simulink model "Model"  (R2020b)
settings: Solver=VariableStepAuto  StartTime=0.0  StopTime=20  MaxStep=0.1  RelTol=1e-1
values from neighbouring files (symbols this model uses):
  D = [0 ... (first row only)    [Data_clean.m]
  g = 9.81    [Data_clean.m]
  k_cart = 0.0113    [Data_clean.m]
  L = 5    [Data_clean.m]
  m = 12000    [Data_clean.m]
  M = 1000    [Data_clean.m]
  Ts = 0.1    [Data_clean.m]
undefined symbols (not defined in the file or in its folder): blk, Discrete, iA, isLTV, lastPcov, lastu, lastx, MDscale, mpc1_plant, MVscale, nCC, nu, nud, nv, nxp, ny, nym, p, RMVscale, Time, ts, uoff, X, xoff, Y, Yscale, Z
libraries: sm_lib x76, mpcsigdimcheck_private x76, nesl_utility x12, ctrlSharedLib x8, simulink_extras x5, mpclib x1
(part 6 of 8)

== system Model/Adaptive MPC Controller2/MPC/MPC Matrix Signal Check U ==
  Input : Inport
  Matrix Dimension Check : S-Function  FunctionName=mpcMatrixSignalCheck  Parameters=blockname, signalname, nrow, ncol, nsteps, isltv  SFunctionDeploymentMode=off  EnableBusSupport=off
  Signal Specification : SignalSpecification  Dimensions=[1 1]
  Output : Outport  VectorParamsAs1DForOutWhenUnconnected=off
  wires:
  Input/1 -> Output/1, Signal Specification/1
  Signal Specification/1 -> Matrix Dimension Check/1

== system Model/Adaptive MPC Controller2/MPC/MPC Matrix Signal Check X ==
  Input : Inport
  Matrix Dimension Check : S-Function  FunctionName=mpcMatrixSignalCheck  Parameters=blockname, signalname, nrow, ncol, nsteps, isltv  SFunctionDeploymentMode=off  EnableBusSupport=off
  Signal Specification : SignalSpecification  Dimensions=[4 1]
  Output : Outport  VectorParamsAs1DForOutWhenUnconnected=off
  wires:
  Input/1 -> Output/1, Signal Specification/1
  Signal Specification/1 -> Matrix Dimension Check/1

== system Model/Adaptive MPC Controller2/MPC/MPC Matrix Signal Check Y ==
  Input : Inport
  Matrix Dimension Check : S-Function  FunctionName=mpcMatrixSignalCheck  Parameters=blockname, signalname, nrow, ncol, nsteps, isltv  SFunctionDeploymentMode=off  EnableBusSupport=off
  Signal Specification : SignalSpecification  Dimensions=[4 1]
  Output : Outport  VectorParamsAs1DForOutWhenUnconnected=off
  wires:
  Input/1 -> Output/1, Signal Specification/1
  Signal Specification/1 -> Matrix Dimension Check/1

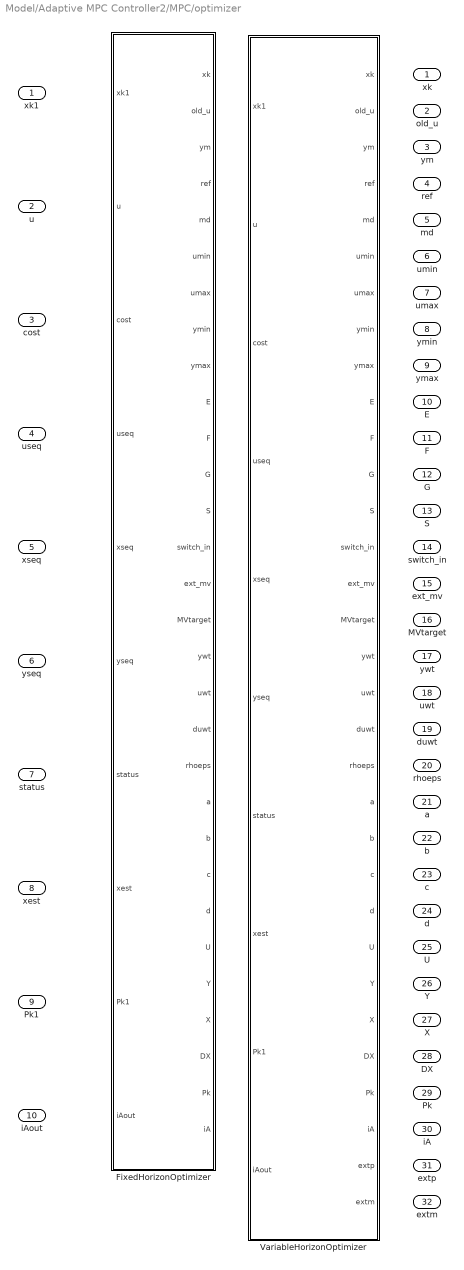
== system Model/Adaptive MPC Controller2/MPC/optimizer ==
  "xk " : Inport
  "old_u " : Inport  Port=2
  "ym " : Inport  Port=3
  "ref " : Inport  Port=4
  "md " : Inport  Port=5
  "umin " : Inport  Port=6
  "umax " : Inport  Port=7
  "ymin " : Inport  Port=8
  "ymax " : Inport  Port=9
  "E " : Inport  Port=10
  "F " : Inport  Port=11
  "G " : Inport  Port=12
  "S " : Inport  Port=13
  "switch_in " : Inport  Port=14
  "ext_mv " : Inport  Port=15
  "MVtarget " : Inport  Port=16
  "ywt " : Inport  Port=17
  "uwt " : Inport  Port=18
  "duwt " : Inport  Port=19
  "rhoeps " : Inport  Port=20
  "a " : Inport  Port=21
  "b " : Inport  Port=22
  "c " : Inport  Port=23
  "d " : Inport  Port=24
  "U " : Inport  Port=25
  "Y " : Inport  Port=26
  "X " : Inport  Port=27
  "DX " : Inport  Port=28
  "Pk " : Inport  Port=29
  "iA " : Inport  Port=30
  extp : Inport  Port=31
  extm : Inport  Port=32
  FixedHorizonOptimizer : MATLAB Function  VariantControl=FixedHorizon
  VariableHorizonOptimizer : MATLAB Function  VariantControl=VariableHorizon
  " xk1" : Outport  VectorParamsAs1DForOutWhenUnconnected=off
  " u" : Outport  Port=2  VectorParamsAs1DForOutWhenUnconnected=off
  " cost" : Outport  Port=3  VectorParamsAs1DForOutWhenUnconnected=off
  " useq" : Outport  Port=4  VectorParamsAs1DForOutWhenUnconnected=off
  " xseq" : Outport  Port=5  VectorParamsAs1DForOutWhenUnconnected=off
  " yseq" : Outport  Port=6  VectorParamsAs1DForOutWhenUnconnected=off
  " status" : Outport  Port=7  VectorParamsAs1DForOutWhenUnconnected=off
  " xest" : Outport  Port=8  VectorParamsAs1DForOutWhenUnconnected=off
  " Pk1" : Outport  Port=9  VectorParamsAs1DForOutWhenUnconnected=off
  " iAout" : Outport  Port=10  VectorParamsAs1DForOutWhenUnconnected=off

== system Model/Adaptive MPC Controller3/MPC/MPC Matrix Signal Check A ==
  Input : Inport
  Matrix Dimension Check : S-Function  FunctionName=mpcMatrixSignalCheck  Parameters=blockname, signalname, nrow, ncol, nsteps, isltv  SFunctionDeploymentMode=off  EnableBusSupport=off
  Signal Specification : SignalSpecification  Dimensions=[4 4]
  Output : Outport  VectorParamsAs1DForOutWhenUnconnected=off
  wires:
  Input/1 -> Output/1, Signal Specification/1
  Signal Specification/1 -> Matrix Dimension Check/1

== system Model/Adaptive MPC Controller3/MPC/MPC Matrix Signal Check B ==
  Input : Inport
  Matrix Dimension Check : S-Function  FunctionName=mpcMatrixSignalCheck  Parameters=blockname, signalname, nrow, ncol, nsteps, isltv  SFunctionDeploymentMode=off  EnableBusSupport=off
  Signal Specification : SignalSpecification  Dimensions=[4 1]
  Output : Outport  VectorParamsAs1DForOutWhenUnconnected=off
  wires:
  Input/1 -> Output/1, Signal Specification/1
  Signal Specification/1 -> Matrix Dimension Check/1

== system Model/Adaptive MPC Controller3/MPC/MPC Matrix Signal Check C ==
  Input : Inport
  Matrix Dimension Check : S-Function  FunctionName=mpcMatrixSignalCheck  Parameters=blockname, signalname, nrow, ncol, nsteps, isltv  SFunctionDeploymentMode=off  EnableBusSupport=off
  Signal Specification : SignalSpecification  Dimensions=[4 4]
  Output : Outport  VectorParamsAs1DForOutWhenUnconnected=off
  wires:
  Input/1 -> Output/1, Signal Specification/1
  Signal Specification/1 -> Matrix Dimension Check/1

== system Model/Adaptive MPC Controller3/MPC/MPC Matrix Signal Check D ==
  Input : Inport
  Matrix Dimension Check : S-Function  FunctionName=mpcMatrixSignalCheck  Parameters=blockname, signalname, nrow, ncol, nsteps, isltv  SFunctionDeploymentMode=off  EnableBusSupport=off
  Signal Specification : SignalSpecification  Dimensions=[4 1]
  Output : Outport  VectorParamsAs1DForOutWhenUnconnected=off
  wires:
  Input/1 -> Output/1, Signal Specification/1
  Signal Specification/1 -> Matrix Dimension Check/1

== system Model/Adaptive MPC Controller3/MPC/MPC Matrix Signal Check DX ==
  Input : Inport
  Matrix Dimension Check : S-Function  FunctionName=mpcMatrixSignalCheck  Parameters=blockname, signalname, nrow, ncol, nsteps, isltv  SFunctionDeploymentMode=off  EnableBusSupport=off
  Signal Specification : SignalSpecification  Dimensions=[4 1]
  Output : Outport  VectorParamsAs1DForOutWhenUnconnected=off
  wires:
  Input/1 -> Output/1, Signal Specification/1
  Signal Specification/1 -> Matrix Dimension Check/1

== system Model/Adaptive MPC Controller3/MPC/MPC Matrix Signal Check U ==
  Input : Inport
  Matrix Dimension Check : S-Function  FunctionName=mpcMatrixSignalCheck  Parameters=blockname, signalname, nrow, ncol, nsteps, isltv  SFunctionDeploymentMode=off  EnableBusSupport=off
  Signal Specification : SignalSpecification  Dimensions=[1 1]
  Output : Outport  VectorParamsAs1DForOutWhenUnconnected=off
  wires:
  Input/1 -> Output/1, Signal Specification/1
  Signal Specification/1 -> Matrix Dimension Check/1

== system Model/Adaptive MPC Controller3/MPC/MPC Matrix Signal Check X ==
  Input : Inport
  Matrix Dimension Check : S-Function  FunctionName=mpcMatrixSignalCheck  Parameters=blockname, signalname, nrow, ncol, nsteps, isltv  SFunctionDeploymentMode=off  EnableBusSupport=off
  Signal Specification : SignalSpecification  Dimensions=[4 1]
  Output : Outport  VectorParamsAs1DForOutWhenUnconnected=off
  wires:
  Input/1 -> Output/1, Signal Specification/1
  Signal Specification/1 -> Matrix Dimension Check/1

== system Model/Adaptive MPC Controller3/MPC/MPC Matrix Signal Check Y ==
  Input : Inport
  Matrix Dimension Check : S-Function  FunctionName=mpcMatrixSignalCheck  Parameters=blockname, signalname, nrow, ncol, nsteps, isltv  SFunctionDeploymentMode=off  EnableBusSupport=off
  Signal Specification : SignalSpecification  Dimensions=[4 1]
  Output : Outport  VectorParamsAs1DForOutWhenUnconnected=off
  wires:
  Input/1 -> Output/1, Signal Specification/1
  Signal Specification/1 -> Matrix Dimension Check/1

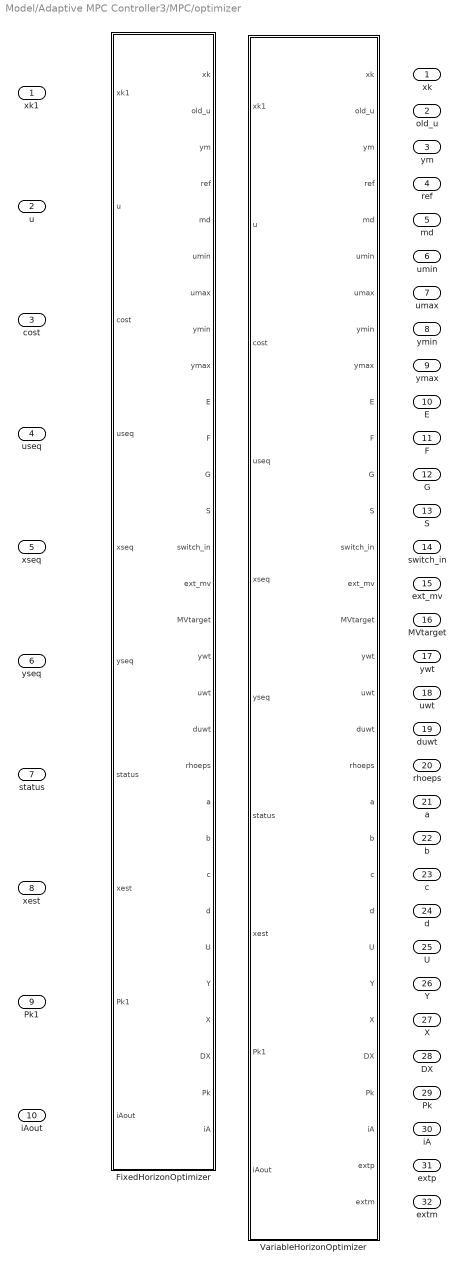
== system Model/Adaptive MPC Controller3/MPC/optimizer ==
  "xk " : Inport
  "old_u " : Inport  Port=2
  "ym " : Inport  Port=3
  "ref " : Inport  Port=4
  "md " : Inport  Port=5
  "umin " : Inport  Port=6
  "umax " : Inport  Port=7
  "ymin " : Inport  Port=8
  "ymax " : Inport  Port=9
  "E " : Inport  Port=10
  "F " : Inport  Port=11
  "G " : Inport  Port=12
  "S " : Inport  Port=13
  "switch_in " : Inport  Port=14
  "ext_mv " : Inport  Port=15
  "MVtarget " : Inport  Port=16
  "ywt " : Inport  Port=17
  "uwt " : Inport  Port=18
  "duwt " : Inport  Port=19
  "rhoeps " : Inport  Port=20
  "a " : Inport  Port=21
  "b " : Inport  Port=22
  "c " : Inport  Port=23
  "d " : Inport  Port=24
  "U " : Inport  Port=25
  "Y " : Inport  Port=26
  "X " : Inport  Port=27
  "DX " : Inport  Port=28
  "Pk " : Inport  Port=29
  "iA " : Inport  Port=30
  extp : Inport  Port=31
  extm : Inport  Port=32
  FixedHorizonOptimizer : MATLAB Function  VariantControl=FixedHorizon
  VariableHorizonOptimizer : MATLAB Function  VariantControl=VariableHorizon
  " xk1" : Outport  VectorParamsAs1DForOutWhenUnconnected=off
  " u" : Outport  Port=2  VectorParamsAs1DForOutWhenUnconnected=off
  " cost" : Outport  Port=3  VectorParamsAs1DForOutWhenUnconnected=off
  " useq" : Outport  Port=4  VectorParamsAs1DForOutWhenUnconnected=off
  " xseq" : Outport  Port=5  VectorParamsAs1DForOutWhenUnconnected=off
  " yseq" : Outport  Port=6  VectorParamsAs1DForOutWhenUnconnected=off
  " status" : Outport  Port=7  VectorParamsAs1DForOutWhenUnconnected=off
  " xest" : Outport  Port=8  VectorParamsAs1DForOutWhenUnconnected=off
  " Pk1" : Outport  Port=9  VectorParamsAs1DForOutWhenUnconnected=off
  " iAout" : Outport  Port=10  VectorParamsAs1DForOutWhenUnconnected=off

== matlab function Model/Plant Model3 ==
  data: u input; A output; x input; B output; C output; D output; U output; Y output; X output; DX output; m input; L input
function [A,B,C,D,U,Y,X,DX] = fcn(u,x,m,L)
% Sample time
Ts = 0.1;

% Model parameters
M = 1000;               % Cart mass, kg
g = 9.81;               % Gravity constant, m/s^2 
k_cart = 0.0113;        % Rolling resistance coefficient   

% Continuos-time model
% Calculated constants
c1 = 1 - m/(m + M);
c2 = -1/(L*(m + M));

A = [-k_cart*(m + M)*g/M    0     0    m*g/M
              1             0     0      0
       k_cart*g/(L*c1)      0     0  -g/(L*c1) 
              0             0     1      0];
 
B = [1/M
      0
    c2/c1
      0];

C = [0 1 0 0
     1 0 0 0
     0 0 0 1
     0 0 1 0];
     
D = [0
     0
     0
     0];
  
% Generate discrete-time model
nx = size(A,1);
nu = size(B,2);
Mr = expm([[A B]*Ts; zeros(nu,nx+nu)]);
A = Mr(1:nx,1:nx);
B = Mr(1:nx,nx+1:nx+nu);

% Nominal conditions for discrete-time plant
X = x;
U = u;
Y = C*x + D*u;
DX = A*x+B*u-x;

== matlab function Model/no_expm1 ==
  data: u input; A output; x input; B output; C output; D output; U output; Y output; X output; DX output; m input; L input
function [A,B,C,D,U,Y,X,DX] = fcn(u,x,m,L)
% Sample time
Ts = 0.1;

% Model parameters
M = 1000;               % Cart mass, kg
g = 9.81;               % Gravity constant, m/s^2 
k_cart = 0.0113;        % Rolling resistance coefficient   

% Continuos-time model
% Calculated constants
c1 = 1 - m/(m + M);
c2 = -1/(L*(m + M));

Ac = [-k_cart*(m + M)*g/M    0     0    m*g/M
              1              0     0      0
       k_cart*g/(L*c1)       0     0  -g/(L*c1) 
              0              0     1      0];
 
Bc = [1/M
       0
     c2/c1
       0];

Cc = [0 1 0 0
      1 0 0 0
      0 0 0 1
      0 0 1 0];
     
Dc = [0
      0
      0
      0];
  
% Generate discrete-time model
nx = size(Ac,1);
nu = size(Bc,2);

% Expm function
X_exp = [[Ac Bc]*Ts; zeros(nu,nx+nu)];
[V_exp,D_exp] = eig(X_exp);
Mr = real(V_exp*diag(exp(diag(D_exp)))/V_exp);
Mr(2,5) = 0;

A = Mr(1:nx,1:nx);
B = Mr(1:nx,nx+1:nx+nu);

% Nominal conditions for discrete-time plant
C = Cc;
D = Dc;

X = x;
U = u;
Y = C*x + D*u;
DX = A*x+B*u-x;

== matlab function Model/Adaptive MPC Controller3/MPC/optimizer/FixedHorizonOptimizer ==
  settings: updateMethod=DISCRETE  sampleTime=ts
  data: xk1 output BlockDataType; xk input BlockDataType; old_u input BlockDataType; ym input BlockDataType; ref input BlockDataType; md input BlockDataType; umin input BlockDataType; umax input BlockDataType; ymin input BlockDataType; ymax input BlockDataType; E input BlockDataType; F input BlockDataType; G input BlockDataType; S input BlockDataType; switch_in input BlockDataType; ext_mv input BlockDataType; MVtarget input BlockDataType; isQP parameter boolean; nx parameter BlockDataType; nxp parameter BlockDataType; nup parameter BlockDataType; nu parameter BlockDataType; ny parameter BlockDataType; degrees parameter BlockDataType; Hinv parameter BlockDataType; Kx parameter BlockDataType; Ku1 parameter BlockDataType; Kut parameter BlockDataType; Kr parameter BlockDataType; Kv parameter BlockDataType; Mlim parameter BlockDataType; Mx parameter BlockDataType; Mu1 parameter BlockDataType; Mv parameter BlockDataType; z_degrees parameter BlockDataType; utarget parameter BlockDataType; p parameter BlockDataType; CustomSolver parameter boolean; CustomSolverCodeGen parameter boolean; UseSuboptimalSolution parameter boolean; UseActiveSetSolver parameter boolean; ASOptions parameter; nxQP parameter BlockDataType; openloopflag parameter boolean; no_umin parameter BlockDataType; no_umax parameter BlockDataType; no_ymin parameter BlockDataType; no_ymax parameter BlockDataType; switch_inport parameter BlockDataType; no_switch parameter BlockDataType; enable_value parameter BlockDataType; return_cost parameter BlockDataType; H parameter BlockDataType; return_mvseq parameter BlockDataType; return_xseq parameter BlockDataType; return_ovseq parameter BlockDataType; Linv parameter BlockDataType; Ac parameter BlockDataType; ywt input BlockDataType; uwt input BlockDataType; duwt input BlockDataType; rhoeps input BlockDataType; isLTV parameter boolean; a input BlockDataType; b input BlockDataType; c input BlockDataType; d input BlockDataType; U input BlockDataType; Y input BlockDataType; X input BlockDataType; DX input BlockDataType; Pk input BlockDataType; iA input boolean; u output BlockDataType; cost output BlockDataType; useq output BlockDataType; xseq output BlockDataType; yseq output BlockDataType; status output BlockDataType; xest output BlockDataType; Pk1 output BlockDataType; no_ywt parameter BlockDataType; no_uwt parameter BlockDataType; no_duwt parameter BlockDataType; no_rhoeps parameter BlockDataType; Wy parameter BlockDataType; Wdu parameter BlockDataType; Jm parameter BlockDataType; SuJm parameter BlockDataType; Su1 parameter BlockDataType; Sx parameter BlockDataType; Hv parameter BlockDataType; Wu parameter BlockDataType; I1 parameter BlockDataType; iAout output boolean; A parameter BlockDataType; C parameter BlockDataType; B parameter BlockDataType; D parameter BlockDataType; Cid parameter BlockDataType; Did parameter BlockDataType; Mrows parameter BlockDataType; nCC parameter BlockDataType; Ecc parameter BlockDataType; Fcc parameter BlockDataType; Scc parameter BlockDataType; Gcc parameter BlockDataType; nv parameter BlockDataType; no_md parameter BlockDataType; no_ref parameter BlockDataType; no_uref parameter BlockDataType; no_mv parameter BlockDataType; RYscale parameter BlockDataType; RMDscale parameter BlockDataType; myindex parameter BlockDataType; xoff parameter BlockDataType; CustomEstimation parameter boolean; mvindex parameter BlockDataType; mdindex parameter BlockDataType; unindex parameter BlockDataType; nxid parameter BlockDataType; Uscale parameter BlockDataType; Yscale parameter BlockDataType; uoff parameter BlockDataType; voff parameter BlockDataType; yoff parameter BlockDataType; myoff parameter BlockDataType; no_cc parameter BlockDataType; IPOptions parameter; RMVscale parameter; m parameter
function [xk1, u, cost, useq, xseq, yseq, status, xest, Pk1, iAout] = fcn(...
            xk, old_u, ym, ref, md, umin, umax, ymin, ymax, E, F, G, S,...
            switch_in, ext_mv, MVtarget, isQP, nx, nxp, nup, ...
            nu, ny, degrees, Hinv, Kx, Ku1, Kut, Kr, Kv, Mlim, ...
            Mx, Mu1, Mv, z_degrees, utarget, p, ...
            CustomSolver, CustomSolverCodeGen, UseSuboptimalSolution, ...
            UseActiveSetSolver, ASOptions, nxQP, openloopflag, ...
            no_umin, no_umax, no_ymin, no_ymax, switch_inport, no_switch, enable_value, ...
            return_cost, H, return_mvseq, return_xseq, return_ovseq, Linv, Ac, ...
            ywt, uwt, duwt, rhoeps, isLTV, a, b, c, d, U, Y, X, DX, Pk, iA, ...
            no_ywt, no_uwt, no_duwt, no_rhoeps,...
            Wy, Wdu, Jm, SuJm, Su1, Sx, Hv, Wu, I1, ...
            A, C, B, D, Cid, Did, Mrows, nCC, Ecc, Fcc, Scc, Gcc, ...
            nv, no_md, no_ref, no_uref, no_mv, RYscale, RMDscale, myindex, ...
            xoff, CustomEstimation, mvindex, mdindex, unindex, nxid, Uscale, Yscale, uoff, voff, yoff, myoff, no_cc, IPOptions, RMVscale, m)
%#codegen
coder.extrinsic('mpcblock_optimizer_double_mex');
coder.extrinsic('mpcblock_optimizer_single_mex');
coder.extrinsic('mpcblock_refmd_double_mex');
coder.extrinsic('mpcblock_refmd_single_mex');

% Constants
isSimulation = coder.target('Sfun') && ~coder.target('RtwForRapid') && ~coder.target('RtwForSim');
isAdaptive = ~isLTV; % isLTV=true forces isAdaptive=false
isDouble = isa(ref,'double');
if isDouble
    DataType = 'double';
else
    DataType = 'single';
end
ZERO = zeros('like',ref);
ONE = ones('like',ref);
hasMD = nv>1;

% Pre-allocate all the MEX block outputs for the simulation mode
%#ok<*NASGU>
if isSimulation
    rseq = zeros(p*ny,1,'like',ref); %#ok<*NASGU>
    vseq = zeros((p+1)*nv,1,'like',ref);
    v = zeros(nv,1,'like',ref);
    xk1 = zeros(nx,1,'like',ref);
    u = zeros(nu,1,'like',ref);
    cost = ZERO;
    useq = zeros(p+1,nu,'like',ref); %#ok<*PREALL>
    status = ONE;
    xest = zeros(nx,1,'like',ref);
    iAout = iA;
end

% Model update
nym = length(myindex);
ai=zeros(nxp,nxp,'like',ref);
bi=zeros(nxp,nup,'like',ref);
ci=zeros(ny,nxp,'like',ref);
di=zeros(ny,nup,'like',ref);

ai(:,:)=a(:,:,1);
bi(:,:)=b(:,:,1);
ci(:,:)=c(:,:,1);
di(:,:)=d(:,:,1);

% Allocate matrices. Must allocate 3D matrix also in Adaptive case,
% otherwise EML code does not compile.
Bu=zeros(nx,nu,p+1,'like',ref);
Bv=zeros(nx,nv,p+1,'like',ref);
Dv=zeros(ny,nv,p+1,'like',ref);
Dvm=zeros(nym,nv,p+1,'like',ref);
Cm=zeros(nym,nx,p+1,'like',ref);
if ~isLTV
    % Adaptive
    [A(:,:,1),C(:,:,1),Bu(:,:,1),Bv(:,:,1),Cm(:,:,1),Dv(:,:,1),Dvm(:,:,1),Qk,Rk,Nk] = mpc_plantupdate(...
        ai,bi,ci,di,A(:,:,1),B(:,:,1),C(:,:,1),D(:,:,1),mvindex,mdindex,unindex,nxp,nup,ny,nv,nxid, ...
        myindex,Uscale,Yscale,Cid,Did);
else
    % Retrieve LTV model
    for i=1:p+1
        ai(1:nxp,1:nxp)=a(:,:,i);
        bi(1:nxp,1:nup)=b(:,:,i);
        ci(1:ny,1:nxp)=c(:,:,i);
        di(1:ny,1:nup)=d(:,:,i);
        [A(:,:,i),C(:,:,i),Bu(:,:,i),Bv(:,:,i),Cm(:,:,i),Dv(:,:,i),Dvm(:,:,i),Qk,Rk,Nk] =...
            mpc_plantupdate(ai,bi,ci,di,A(:,:,i),B(:,:,i),C(:,:,i),D(:,:,i),mvindex,mdindex,unindex,nxp,nup,ny,nv,nxid, ...
            myindex,Uscale,Yscale,Cid,Did);
    end
end

% Offset update together with Mlim, utarget, Bv and Dv values
[Mlim, utarget, uoff, voff, yoff, myoff, xoff, Bv, Dv] = ...
    mpc_updateFromNominal(isAdaptive,isQP,p,Mlim,Mrows,...
       U,Uscale,uoff,mvindex,voff,mdindex,utarget,nu,nv-1,...
       Y,Yscale,yoff,myoff,myindex,ny,...
       X,xoff,nxp,DX,A,Bu,Bv,C,Dv,nCC);

% Remove last u offset
old_u = old_u - uoff;       

% Get reference and MD signals -- accounting for previewing
if isSimulation
    if isDouble
        [rseq, vseq, v] = mpcblock_refmd_double_mex(ref,md,nv,ny,p,yoff,voff,no_md,no_ref,openloopflag, RYscale, RMDscale);
    else
        [rseq, vseq, v] = mpcblock_refmd_single_mex(ref,md,nv,ny,p,yoff,voff,no_md,no_ref,openloopflag, RYscale, RMDscale);        
    end
else
    % When doing code generation, use M code directly
    [rseq, vseq, v] = mpcblock_refmd(ref,md,nv,ny,p,yoff,voff,no_md,no_ref,openloopflag, RYscale, RMDscale);
end

% External MV override.  
% NOTE: old_u and ext_mv input signals are dimensionless and offset-free.
if no_mv==ONE
    % no external mv: old_u is the optimal u[k-1] from last_mv
    delmv = zeros(nu,1,'like',ref);
else
    % has external mv: old_u is the external u[k-1]
    ext_mv = ext_mv - uoff;     % bias correction
    delmv = ext_mv - old_u;
    old_u = ext_mv;
end

% Obtain x[k|k]
xk = xk - xoff;     % Remove offset
if CustomEstimation==ONE
    % Input is x(k|k)
    xest = xk;
else
    % Calculate gain matrices, and perform measurement update.
    Kinv = eye(nym,'like',ref)/(Cm(:,:,1)*Pk*Cm(:,:,1)' + Rk);
    L = (A(:,:,1)*Pk*Cm(:,:,1)' + Nk)*Kinv;
    M = Pk*Cm(:,:,1)'*Kinv;
    % LTVKF state estimation.
    % Scale measured output and remove offset.
    ym = ym.*RYscale(myindex) - myoff;
    % Correct x(k|k-1) for possible external mv override.
    % NOTE:  Offset was removed from x[k|k-1] at k=0.
    xk = xk + Bu(:,:,1)*delmv;
    % Measurement upate to x(k|k)
    ym_est = Cm(:,:,1)*xk + Dvm(:,:,1)*v;
    y_innov = ym - ym_est;
    xest = xk + M*y_innov;
end

% Real-time MV target override
% Note: utargetValue is a vector length p*nu.  
if no_uref==ONE
    % no external utarget
    utargetValue = utarget;
else
    % Define constant targets for the entire horizon.
    MVtarget = MVtarget - uoff;         % Bias correction
    utargetValue = reshape(MVtarget(:,ones(p,1)),nu*p,1);
end

% Real-time custom constraint override (scaled E/F/S)
if no_cc~=ONE
    Ecc = E;
    Fcc = F;
    Gcc = G;
    if nv>1
        Scc = S;
    end
end

return_sequence = (return_mvseq || return_xseq || return_ovseq)*ONE;
if isSimulation
    if isDouble
        [u, cost, useq, status, iAout] = mpcblock_optimizer_double_mex(...
            rseq, vseq, umin, umax, ymin, ymax, switch_in, xest, old_u, iA, ...
            isQP, nu, ny, degrees, Hinv, Kx, Ku1, Kut, Kr, Kv, Mlim, ...
            Mx, Mu1, Mv, z_degrees, utargetValue, p, uoff, voff, yoff, ...
            CustomSolver, false, UseSuboptimalSolution, ...
            UseActiveSetSolver, ASOptions, IPOptions, nxQP, openloopflag, ...
            no_umin, no_umax, no_ymin, no_ymax, no_cc, switch_inport, ...
            no_switch, enable_value, return_cost, H, return_sequence, Linv, Ac, ...
            ywt, uwt, duwt, rhoeps, no_ywt, no_uwt, no_duwt, no_rhoeps,...
            Wy, Wdu, Jm, SuJm, Su1, Sx, Hv, Wu, I1, ...
            isAdaptive, isLTV, A, Bu, Bv, C, Dv, ...
            Mrows, nCC, Ecc, Fcc, Scc, Gcc, RYscale, RMVscale, m);    
    else
        [u, cost, useq, status, iAout] = mpcblock_optimizer_single_mex(...
            rseq, vseq, umin, umax, ymin, ymax, switch_in, xest, old_u, iA, ...
            isQP, nu, ny, degrees, Hinv, Kx, Ku1, Kut, Kr, Kv, Mlim, ...
            Mx, Mu1, Mv, z_degrees, utargetValue, p, uoff, voff, yoff, ...
            CustomSolver, false, UseSuboptimalSolution, ...
            UseActiveSetSolver, ASOptions, IPOptions, nxQP, openloopflag, ...
            no_umin, no_umax, no_ymin, no_ymax, no_cc, switch_inport, ...
            no_switch, enable_value, return_cost, H, return_sequence, Linv, Ac, ...
            ywt, uwt, duwt, rhoeps, no_ywt, no_uwt, no_duwt, no_rhoeps,...
            Wy, Wdu, Jm, SuJm, Su1, Sx, Hv, Wu, I1, ...
            isAdaptive, isLTV, A, Bu, Bv, C, Dv, ...
            Mrows, nCC, Ecc, Fcc, Scc, Gcc, RYscale, RMVscale, m);    
    end
else
    % When doing code generation, use M code directly
        [u, cost, useq, status, iAout] = mpcblock_optimizer(...
            rseq, vseq, umin, umax, ymin, ymax, switch_in, xest, old_u, iA, ...
            isQP, nu, ny, degrees, Hinv, Kx, Ku1, Kut, Kr, Kv, Mlim, ...
            Mx, Mu1, Mv, z_degrees, utargetValue, p, uoff, voff, yoff, ...
            false, CustomSolverCodeGen, UseSuboptimalSolution, ...
            UseActiveSetSolver, ASOptions, IPOptions, nxQP, openloopflag, ...
            no_umin, no_umax, no_ymin, no_ymax, no_cc, switch_inport, ...
            no_switch, enable_value, return_cost, H, return_sequence, Linv, Ac, ...
            ywt, uwt, duwt, rhoeps, no_ywt, no_uwt, no_duwt, no_rhoeps,...
            Wy, Wdu, Jm, SuJm, Su1, Sx, Hv, Wu, I1, ...
            isAdaptive, isLTV, A, Bu, Bv, C, Dv, ...
            Mrows, nCC, Ecc, Fcc, Scc, Gcc, RYscale, RMVscale, m);    
end

if return_xseq || return_ovseq
    [yseq, xseq] = mpc_computeSequence(isLTV, xest, useq, vseq, uoff, yoff, xoff, p, ny, nxQP, nv, A, Bu, Bv, C, Dv);
else
    yseq = zeros(p+1,ny,'like',rseq);
    xseq = zeros(p+1,nxQP,'like',rseq);
end

if CustomEstimation==ONE
    xk1 = zeros(nx,1,'like',ref);
    Pk1 = Pk;
else
    % LTVKF state and covariance update
    xk1 = A(:,:,1)*xk + Bu(:,:,1)*(u - uoff) + Bv(:,:,1)*v + L*y_innov;
    Pk1 = A(:,:,1)*Pk*A(:,:,1)' - (A(:,:,1)*Pk*Cm(:,:,1)' + Nk)*L' + Qk;
    Pk1 = 0.5*(Pk1 + Pk1'); % guarantee symmetric for numerical stability
end
xk1 = xk1 + xoff;   % Updated state must include offset

% return xest in original value
xest = xest + xoff;

== matlab function Model/Adaptive MPC Controller3/MPC/optimizer/VariableHorizonOptimizer ==
  settings: updateMethod=DISCRETE  sampleTime=ts
  data: xk1 output BlockDataType; xk input BlockDataType; old_u input BlockDataType; ym input BlockDataType; ref input BlockDataType; md input BlockDataType; umin input BlockDataType; umax input BlockDataType; ymin input BlockDataType; ymax input BlockDataType; E input BlockDataType; F input BlockDataType; G input BlockDataType; S input BlockDataType; switch_in input BlockDataType; ext_mv input BlockDataType; MVtarget input BlockDataType; isQP parameter boolean; nx parameter BlockDataType; nxp parameter BlockDataType; nup parameter BlockDataType; nu parameter BlockDataType; ny parameter BlockDataType; degrees parameter BlockDataType; Mlim parameter BlockDataType; Mx parameter BlockDataType; Mu1 parameter BlockDataType; Mv parameter BlockDataType; utarget parameter BlockDataType; p parameter BlockDataType; CustomSolver parameter boolean; CustomSolverCodeGen parameter boolean; UseSuboptimalSolution parameter boolean; UseActiveSetSolver parameter boolean; nxQP parameter BlockDataType; openloopflag parameter boolean; no_umin parameter BlockDataType; no_umax parameter BlockDataType; no_ymin parameter BlockDataType; no_ymax parameter BlockDataType; switch_inport parameter BlockDataType; no_switch parameter BlockDataType; enable_value parameter BlockDataType; return_cost parameter BlockDataType; H parameter BlockDataType; return_mvseq parameter BlockDataType; return_xseq parameter BlockDataType; return_ovseq parameter BlockDataType; Ac parameter BlockDataType; ywt input BlockDataType; uwt input BlockDataType; duwt input BlockDataType; rhoeps input BlockDataType; isLTV parameter boolean; a input BlockDataType; b input BlockDataType; c input BlockDataType; d input BlockDataType; U input BlockDataType; Y input BlockDataType; X input BlockDataType; DX input BlockDataType; Pk input BlockDataType; iA input boolean; extp input BlockDataType; extm input BlockDataType; u output BlockDataType; cost output BlockDataType; useq output BlockDataType; xseq output BlockDataType; yseq output BlockDataType; status output BlockDataType; xest output BlockDataType; Pk1 output BlockDataType; no_ywt parameter BlockDataType; no_uwt parameter BlockDataType; no_duwt parameter BlockDataType; no_rhoeps parameter BlockDataType; Wy parameter BlockDataType; Wdu parameter BlockDataType; Wu parameter BlockDataType; iAout output boolean; A parameter BlockDataType; C parameter BlockDataType; B parameter BlockDataType; D parameter BlockDataType; Cid parameter BlockDataType; Did parameter BlockDataType; Mrows parameter BlockDataType; nCC parameter BlockDataType; Ecc parameter BlockDataType; Fcc parameter BlockDataType; Scc parameter BlockDataType; Gcc parameter BlockDataType; nv parameter BlockDataType; no_md parameter BlockDataType; no_ref parameter BlockDataType; no_uref parameter BlockDataType; no_mv parameter BlockDataType; RYscale parameter BlockDataType; RMDscale parameter BlockDataType; myindex parameter BlockDataType; xoff parameter BlockDataType; CustomEstimation parameter boolean; mvindex parameter BlockDataType; mdindex parameter BlockDataType; unindex parameter BlockDataType; nxid parameter BlockDataType; Uscale parameter BlockDataType; Yscale parameter BlockDataType; uoff parameter BlockDataType; voff parameter BlockDataType; yoff parameter BlockDataType; myoff parameter BlockDataType; no_cc parameter BlockDataType; p0 parameter; ASOptions parameter; IPOptions parameter; RMVscale parameter; m parameter
function [xk1, u, cost, useq, xseq, yseq, status, xest, Pk1, iAout] = fcn(...
            xk, old_u, ym, ref, md, umin, umax, ymin, ymax, E, F, G, S,...
            switch_in, ext_mv, MVtarget, isQP, nx, nxp, nup, ...
            nu, ny, degrees, Mlim, Mx, Mu1, Mv, utarget, p, ...
            CustomSolver, CustomSolverCodeGen, UseSuboptimalSolution, ...
            UseActiveSetSolver, nxQP, openloopflag, ...
            no_umin, no_umax, no_ymin, no_ymax, switch_inport, no_switch, enable_value, ...
            return_cost, H, return_mvseq, return_xseq, return_ovseq, Ac, ...
            ywt, uwt, duwt, rhoeps, isLTV, a, b, c, d, U, Y, X, DX, Pk, iA, extp, extm, ...
            no_ywt, no_uwt, no_duwt, no_rhoeps,...
            Wy, Wdu, Wu, A, C, B, D, Cid, Did, Mrows, nCC, Ecc, Fcc, Scc, Gcc, ...
            nv, no_md, no_ref, no_uref, no_mv, RYscale, RMDscale, myindex, ...
            xoff, CustomEstimation, mvindex, mdindex, unindex, nxid, Uscale, Yscale, uoff, voff, yoff, myoff, no_cc, ...
            p0, ASOptions, IPOptions, RMVscale, m)
%#codegen
coder.extrinsic('mpcblock_optimizerPM_double_mex');
coder.extrinsic('mpcblock_optimizerPM_single_mex');
coder.extrinsic('mpcblock_refmd_double_mex');
coder.extrinsic('mpcblock_refmd_single_mex');

% The following is for DEBUG:
%%%%%%%%%%%%%%%
% coder.extrinsic('mpcblock_optimizerPM');
%%%%%%%%%%%%%%%

% Constants
isSimulation = coder.target('Sfun') && ~coder.target('RtwForRapid') && ~coder.target('RtwForSim');
isAdaptive = ~isLTV; % isLTV=true forces isAdaptive=false
isDouble = isa(ref,'double');
if isDouble
    DataType = 'double';
else
    DataType = 'single';
end
ZERO = zeros('like',ref);
ONE = ones('like',ref);
hasMD = nv>1;

% Keep output arguments related to prediction horizon (useq,xseq,yseq) of 
% size pmax, so that they don't change dimension in case extp varies. 
% Here pmax = input parameter 'p'.

% Pre-allocate all the MEX block outputs for the simulation mode
%#ok<*NASGU>
if isSimulation
    rseq = zeros(extp*ny,1,'like',ref); %#ok<*NASGU>
    vseq = zeros((extp+1)*nv,1,'like',ref);
    v = zeros(nv,1,'like',ref);
    xk1 = zeros(nx,1,'like',ref);
    u = zeros(nu,1,'like',ref);
    cost = ZERO;
    useq = zeros(p+1,nu,'like',ref); %#ok<*PREALL>
    status = ONE;
    xest = zeros(nx,1,'like',ref);
    iAout = iA;
end

% Model update
nym = length(myindex);
ai=zeros(nxp,nxp,'like',ref);
bi=zeros(nxp,nup,'like',ref);
ci=zeros(ny,nxp,'like',ref);
di=zeros(ny,nup,'like',ref);

ai(:,:)=a(:,:,1);
bi(:,:)=b(:,:,1);
ci(:,:)=c(:,:,1);
di(:,:)=d(:,:,1);

% Allocate matrices. Must allocate 3D matrix also in Adaptive case,
% otherwise EML code does not compile.
Bu=zeros(nx,nu,extp+1,'like',ref);
Bv=zeros(nx,nv,extp+1,'like',ref);
Dv=zeros(ny,nv,extp+1,'like',ref);
Dvm=zeros(nym,nv,extp+1,'like',ref);
Cm=zeros(nym,nx,extp+1,'like',ref);
if ~isLTV
    % Adaptive
    [A(:,:,1),C(:,:,1),Bu(:,:,1),Bv(:,:,1),Cm(:,:,1),Dv(:,:,1),Dvm(:,:,1),Qk,Rk,Nk] = mpc_plantupdate(...
        ai,bi,ci,di,A(:,:,1),B(:,:,1),C(:,:,1),D(:,:,1),mvindex,mdindex,unindex,nxp,nup,ny,nv,nxid, ...
        myindex,Uscale,Yscale,Cid,Did);
else
    % Retrieve LTV model
    for i=1:extp+1
        ai(1:nxp,1:nxp)=a(:,:,i);
        bi(1:nxp,1:nup)=b(:,:,i);
        ci(1:ny,1:nxp)=c(:,:,i);
        di(1:ny,1:nup)=d(:,:,i);
        [A(:,:,i),C(:,:,i),Bu(:,:,i),Bv(:,:,i),Cm(:,:,i),Dv(:,:,i),Dvm(:,:,i),Qk,Rk,Nk] =...
            mpc_plantupdate(ai,bi,ci,di,A(:,:,i),B(:,:,i),C(:,:,i),D(:,:,i),mvindex,mdindex,unindex,nxp,nup,ny,nv,nxid, ...
            myindex,Uscale,Yscale,Cid,Did);
    end
end

% Offset update together with Mlim, utarget, Bv and Dv values
[Mlim, utarget, uoff, voff, yoff, myoff, xoff, Bv, Dv] = ...
    mpc_updateFromNominal(isAdaptive,isQP,p0,Mlim,Mrows,...
       U,Uscale,uoff,mvindex,voff,mdindex,utarget,nu,nv-1,...
       Y,Yscale,yoff,myoff,myindex,ny,...
       X,xoff,nxp,DX,A,Bu,Bv,C,Dv,nCC);

% Remove last u offset
old_u = old_u - uoff;       

% Get reference and MD signals -- accounting for previewing
if isSimulation
    if isDouble
        %%%%%%%%%%%%%%%%%%%%%%%%%%%%%%%%%%%%%%%%%%%%%
        %%%%%% TEMPORARILY DISABLE MEX FILE %%%%%%%%%
        %%%%%%%%%%%%%%%%%%%%%%%%%%%%%%%%%%%%%%%%%%%%%
        [rseq, vseq, v] = mpcblock_refmd_double_mex(ref,md,nv,ny,extp,yoff,voff,no_md,no_ref,openloopflag, RYscale, RMDscale);
        %[rseq, vseq, v] = mpcblock_refmd(ref,md,nv,ny,extp,yoff,voff,no_md,no_ref,openloopflag, RYscale, RMDscale);
    else
        %%%%%%%%%%%%%%%%%%%%%%%%%%%%%%%%%%%%%%%%%%%%%
        %%%%%% TEMPORARILY DISABLE MEX FILE %%%%%%%%%
        %%%%%%%%%%%%%%%%%%%%%%%%%%%%%%%%%%%%%%%%%%%%%
        [rseq, vseq, v] = mpcblock_refmd_single_mex(ref,md,nv,ny,extp,yoff,voff,no_md,no_ref,openloopflag, RYscale, RMDscale);        
        %[rseq, vseq, v] = mpcblock_refmd(ref,md,nv,ny,extp,yoff,voff,no_md,no_ref,openloopflag, RYscale, RMDscale);        
    end
else
    % When doing code generation, use M code directly
    [rseq, vseq, v] = mpcblock_refmd(ref,md,nv,ny,extp,yoff,voff,no_md,no_ref,openloopflag, RYscale, RMDscale);
end

% External MV override.  
% NOTE: old_u and ext_mv input signals are dimensionless and offset-free.
if no_mv==ONE
    % no external mv: old_u is the optimal u[k-1] from last_mv
    delmv = zeros(nu,1,'like',ref);
else
    % has external mv: old_u is the external u[k-1]
    ext_mv = ext_mv - uoff;     % bias correction
    delmv = ext_mv - old_u;
    old_u = ext_mv;
end

% Obtain x[k|k]
xk = xk - xoff;     % Remove offset
if CustomEstimation==ONE
    % Input is x(k|k)
    xest = xk;
else
    % Calculate gain matrices, and perform measurement update.
    Kinv = eye(nym,'like',ref)/(Cm(:,:,1)*Pk*Cm(:,:,1)' + Rk);
    L = (A(:,:,1)*Pk*Cm(:,:,1)' + Nk)*Kinv;
    M = Pk*Cm(:,:,1)'*Kinv;
    % LTVKF state estimation.
    % Scale measured output and remove offset.
    ym = ym.*RYscale(myindex) - myoff;
    % Correct x(k|k-1) for possible external mv override.
    % NOTE:  Offset was removed from x[k|k-1] at k=0.
    xk = xk + Bu(:,:,1)*delmv;
    % Measurement upate to x(k|k)
    ym_est = Cm(:,:,1)*xk + Dvm(:,:,1)*v;
    y_innov = ym - ym_est;
    xest = xk + M*y_innov;
end

% Real-time MV target override
% Note: utargetValue is a vector length p*nu.  
if no_uref==ONE
    % no external utarget
    utargetValue = utarget;
else
    % Define constant targets for the entire horizon.
    MVtarget = MVtarget - uoff;         % Bias correction
    utargetValue = reshape(MVtarget(:,ones(p,1)),nu*p,1);
end

% Real-time custom constraint override (scaled E/F/S)
if no_cc~=ONE
    Ecc = E;
    Fcc = F;
    Gcc = G;
    if nv>1
        Scc = S;
    end
end

return_sequence = (return_mvseq || return_xseq || return_ovseq)*ONE;

if numel(extm) > 1
    nMoves = numel(extm)*nu;
    %extm(end) = extp - sum(extm(1:end-1));
else
    nMoves = extm*nu;
    %extm = [ones(1,extm-1), extp-extm+1];
end
extdegrees=nMoves+isQP;
extz_degrees = zeros(extdegrees,1,'like',ref);

% The following is for DEBUG:
%%%%%%%%%%%%%%%
% u=zeros(nu,1,'like',ref);
% cost=ZERO;
% useq1=zeros(p+1,nu,'like',ref);
% status=ZERO;
% iAout=false(size(iA));
%%%%%%%%%%%%%%%

if isSimulation
    if isDouble
        %%%%%%%%%%%%%%%%%%%%%%%%%%%%%%%%%%%%%%%%%%%%%
        %%%%%% TEMPORARILY DISABLE MEX FILE %%%%%%%%%
        %%%%%%%%%%%%%%%%%%%%%%%%%%%%%%%%%%%%%%%%%%%%%
        %[u, cost, useq1, status, iAout] = mpcblock_optimizerPM(...
        [u, cost, useq1, status, iAout] = mpcblock_optimizerPM_double_mex(...
            rseq, vseq, umin, umax, ymin, ymax, switch_in, xest, old_u, iA, isQP, nu, ny, ...
            Mlim, Mx, Mu1, Mv, utargetValue, extp, extm, uoff, voff, yoff, ...
            CustomSolver, false, UseSuboptimalSolution, ...
            UseActiveSetSolver, ASOptions, IPOptions, nxQP, openloopflag,...
            no_umin, no_umax, no_ymin, no_ymax, switch_inport,...
            no_switch, enable_value, return_cost, H, return_sequence, Ac,...
            ywt, uwt, duwt, rhoeps, no_ywt, no_uwt, no_duwt, no_rhoeps,...
            Wy, Wdu, Wu, isLTV, A, Bu, Bv, C, Dv,...
            Mrows, nCC, Ecc, Fcc, Scc, Gcc,...
            RYscale, RMVscale, m, p0, degrees, p);    
    else
        %%%%%%%%%%%%%%%%%%%%%%%%%%%%%%%%%%%%%%%%%%%%%
        %%%%%% TEMPORARILY DISABLE MEX FILE %%%%%%%%%
        %%%%%%%%%%%%%%%%%%%%%%%%%%%%%%%%%%%%%%%%%%%%%
        %[u, cost, useq1, status, iAout] = mpcblock_optimizerPM(...
        [u, cost, useq1, status, iAout] = mpcblock_optimizerPM_single_mex(...
            rseq, vseq, umin, umax, ymin, ymax, switch_in, xest, old_u, iA, ...
            isQP, nu, ny, Mlim, Mx, Mu1, Mv, utargetValue, extp, extm, uoff, voff, yoff, ...
            CustomSolver, false, UseSuboptimalSolution, ...
            UseActiveSetSolver, ASOptions, IPOptions, nxQP, openloopflag, ...
            no_umin, no_umax, no_ymin, no_ymax, switch_inport, ...
            no_switch, enable_value, return_cost, H, return_sequence, Ac, ...
            ywt, uwt, duwt, rhoeps, no_ywt, no_uwt, no_duwt, no_rhoeps,...
            Wy, Wdu, Wu, isLTV, A, Bu, Bv, C, Dv, ...
            Mrows, nCC, Ecc, Fcc, Scc, Gcc, ...
            RYscale, RMVscale, m, p0, degrees, p);    
    end
else
    % When doing code generation, use M code directly
        [u, cost, useq1, status, iAout] = mpcblock_optimizerPM(...
            rseq, vseq, umin, umax, ymin, ymax, switch_in, xest, old_u, iA, ...
            isQP, nu, ny, Mlim, Mx, Mu1, Mv, utargetValue, extp, extm, uoff, voff, yoff, ...
            false, CustomSolverCodeGen, UseSuboptimalSolution, ...
            UseActiveSetSolver, ASOptions, IPOptions, nxQP, openloopflag, ...
            no_umin, no_umax, no_ymin, no_ymax, switch_inport, ...
            no_switch, enable_value, return_cost, H, return_sequence, Ac, ...
            ywt, uwt, duwt, rhoeps, no_ywt, no_uwt, no_duwt, no_rhoeps,...
            Wy, Wdu, Wu, isLTV, A, Bu, Bv, C, Dv, ...
            Mrows, nCC, Ecc, Fcc, Scc, Gcc, ...
            RYscale, RMVscale, m, p0, degrees, p);
end

% Add missing zeros in useq
useq = zeros(p+1,nu,'like',rseq);
for k=1:p+1
    if k<=extp+1
        for i=1:nu
            useq(k,i)=useq1(k,i);
        end
    end
end

if return_xseq || return_ovseq
    [yseq, xseq] = mpc_computeSequence(isLTV, xest, useq, vseq, uoff, yoff, xoff, extp, ny, nxQP, nv, A, Bu, Bv, C, Dv);
else
    yseq = zeros(p+1,ny,'like',rseq);
    xseq = zeros(p+1,nxQP,'like',rseq);
end

if CustomEstimation==ONE
    xk1 = zeros(nx,1,'like',ref);
    Pk1 = Pk;
else
    % LTVKF state and covariance update
    xk1 = A(:,:,1)*xk + Bu(:,:,1)*(u - uoff) + Bv(:,:,1)*v + L*y_innov;
    Pk1 = A(:,:,1)*Pk*A(:,:,1)' - (A(:,:,1)*Pk*Cm(:,:,1)' + Nk)*L' + Qk;
    Pk1 = 0.5*(Pk1 + Pk1'); % guarantee symmetric for numerical stability
end
xk1 = xk1 + xoff;   % Updated state must include offset

% return xest in original value
xest = xest + xoff;

== matlab function Model/Plant Model4 ==
  data: u input; A output; x input; B output; C output; D output; U output; Y output; X output; DX output; m input; L input
function [A,B,C,D,U,Y,X,DX] = fcn(u,x,m,L)
% Sample time
Ts = 0.1;

% Model parameters
M = 1000;               % Cart mass, kg
g = 9.81;               % Gravity constant, m/s^2 
k_cart = 0.0113;        % Rolling resistance coefficient   

% Continuos-time model
% Calculated constants
c1 = 1 - m/(m + M);
c2 = -1/(L*(m + M));

A = [-k_cart*(m + M)*g/M    0     0    m*g/M
              1             0     0      0
       k_cart*g/(L*c1)      0     0  -g/(L*c1) 
              0             0     1      0];
 
B = [1/M
      0
    c2/c1
      0];

C = [0 1 0 0
     1 0 0 0
     0 0 0 1
     0 0 1 0];
     
D = [0
     0
     0
     0];
  
% Generate discrete-time model
nx = size(A,1);
nu = size(B,2);
Mr = expm([[A B]*Ts; zeros(nu,nx+nu)]);
A = Mr(1:nx,1:nx);
B = Mr(1:nx,nx+1:nx+nu);

% Nominal conditions for discrete-time plant
X = x;
U = u;
Y = C*x + D*u;
DX = A*x+B*u-x;

== matlab function Model/Plant Model5 ==
  data: u input; A output; x input; B output; C output; D output; U output; Y output; X output; DX output; m input; L input
function [A,B,C,D,U,Y,X,DX] = fcn(u,x,m,L)
% Sample time
Ts = 0.1;

% Model parameters
M = 1000;               % Cart mass, kg
g = 9.81;               % Gravity constant, m/s^2 
k_cart = 0.0113;        % Rolling resistance coefficient   

% Continuos-time model
% Calculated constants
c1 = 1 - m/(m + M);
c2 = -1/(L*(m + M));

A = [-k_cart*(m + M)*g/M    0     0    m*g/M
              1             0     0      0
       k_cart*g/(L*c1)      0     0  -g/(L*c1) 
              0             0     1      0];
 
B = [1/M
      0
    c2/c1
      0];

C = [0 1 0 0
     1 0 0 0
     0 0 0 1
     0 0 1 0];
     
D = [0
     0
     0
     0];
  
% Generate discrete-time model
nx = size(A,1);
nu = size(B,2);
Mr = expm([[A B]*Ts; zeros(nu,nx+nu)]);
A = Mr(1:nx,1:nx);
B = Mr(1:nx,nx+1:nx+nu);

% Nominal conditions for discrete-time plant
X = x;
U = u;
Y = C*x + D*u;
DX = A*x+B*u-x;
